simulink model "restapi_station2_task"  (Simulink 3.00)
undefined symbols (not defined in the file): application, json
libraries: mathlib x4, stringlib x2, analoglib x1, speclib x1

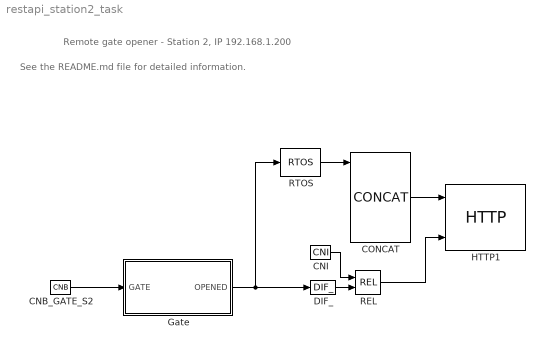
== system restapi_station2_task ==
  note: See the README.md file for detailed information.
  note: Remote gate opener - Station 2, IP 192.168.1.200
  CNB_GATE_S2 : mathlib/CNB  YCN=off
  CNI : mathlib/CNI  icn=0
  CONCAT : stringlib/CONCAT  ptrn="{ \"v\": %1}"  nmax=0
  DIF_ : mathlib/DIF_
  Gate : Subsystem
      mask Type: REX sequence
  HTTP1 : speclib/HTTP  url=http://192.168.1.100:8008/api/tasks/restapi_station1_task/CNB_OPENED:YCN  method=2  VERIFY=off  postmime=application/json  acceptmime=application/json  timeout=5  BLOCKING=off  nmax=0  postmax=256  datamax=1024
  REL : mathlib/REL  irel=2: inequality (!=)
  RTOS : stringlib/RTOS  prec=0  mode=1
  wires:
  CNB_GATE_S2/1 -> Gate/1(GATE)
  CNI/1 -> REL/1
  CONCAT/1 -> HTTP1/1
  DIF_/1 -> REL/2
  Gate/1(OPENED) -> DIF_/1, RTOS/1
  REL/1 -> HTTP1/3
  RTOS/1 -> CONCAT/1

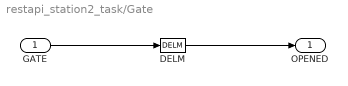
== system restapi_station2_task/Gate ==
  GATE : Inport  Port=1
  DELM : analoglib/DELM  del=5  nmax=100
  OPENED : Outport  Port=1
  wires:
  DELM/1 -> OPENED/1
  GATE/1 -> DELM/1
